simulink model "ch5example2"  (Simulink 5.0)
settings: Solver=ode5  StartTime=0.0  StopTime=0.02  FixedStep=6.23e-8  RelTol=1e-3
values from neighbouring files (symbols this model uses):
  sigma2 = P/SNR_in(k)    [ch5example2prg1.m]
libraries: dsparch4 x6, dspbuff3 x1, dspstat3 x1, dspmathops x1
settings Model: LastModifiedBy=shaoyubin

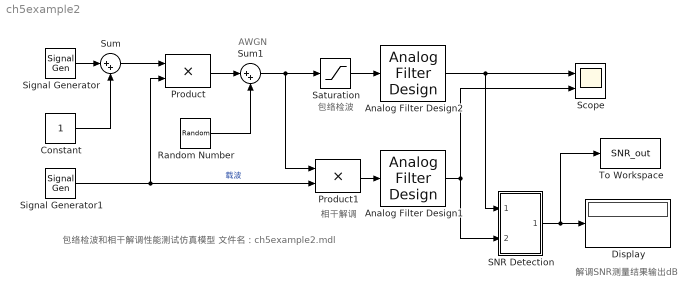
== system ch5example2 ==
  note: 包络检波和相干解调性能测试仿真模型
      | 文件名：ch5example2.mdl
  note: AWGN
  note: 解调SNR测量结果输出dB
  note: 包络检波
  note: 相干解调
  Analog Filter Design1 : dsparch4/Analog Filter Design  method=Butterworth  filttype=Lowpass  N=2  Wlo=2*pi*6e3  Whi=80  Rp=2  Rs=40
  Analog Filter Design2 : dsparch4/Analog Filter Design  method=Butterworth  filttype=Lowpass  N=2  Wlo=2*pi*6e3  Whi=80  Rp=2  Rs=40
  Constant : Constant
  Display : Display
  Product : Product  SaturateOnIntegerOverflow=on
  Product1 : Product  SaturateOnIntegerOverflow=on
  Random Number : RandomNumber  Variance=sigma2  SampleTime=6.23e-8
  SNR Detection : Subsystem
  Saturation : Saturate  UpperLimit=inf  LowerLimit=0
  Scope : Scope  NumInputPorts=2
      settings: TimeRange=0.005  YMin=0~0  YMax=1~1
  Signal Generator : SignalGenerator  Amplitude=0.3*1  Frequency=1000
  Signal Generator1 : SignalGenerator  Frequency=1000e3
  Sum : Sum  Inputs=|++  SaturateOnIntegerOverflow=on
  Sum1 : Sum  Inputs=|++  SaturateOnIntegerOverflow=on
  To Workspace : ToWorkspace  VariableName=SNR_out  SampleTime=-1  SaveFormat=Array
      settings: MaxDataPoints=1
  wires:
  Constant/1 -> Sum/2
  Signal Generator/1 -> Sum/1
  Sum/1 -> Product/1
  Signal Generator1/1 -> Product/2, Product1/2  "载波"
  Product/1 -> Sum1/1
  Random Number/1 -> Sum1/2
  Sum1/1 -> Saturation/1, Product1/1
  Saturation/1 -> Analog Filter Design2/1
  Analog Filter Design2/1 -> SNR Detection/1(In1), Scope/1
  Product1/1 -> Analog Filter Design1/1
  Analog Filter Design1/1 -> SNR Detection/2(In2), Scope/2
  SNR Detection/1(Out1) -> Display/1, To Workspace/1

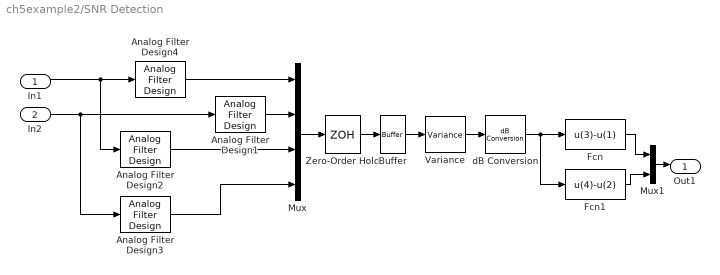
== system ch5example2/SNR Detection ==
  In1 : Inport
  In2 : Inport  Port=2
  Analog Filter Design1 : dsparch4/Analog Filter Design  method=Butterworth  filttype=Bandstop  N=2  Wlo=2*pi*(1e3-100)  Whi=2*pi*(1e3+100)  Rp=2  Rs=40
  Analog Filter Design2 : dsparch4/Analog Filter Design  method=Butterworth  filttype=Bandpass  N=2  Wlo=2*pi*(1e3-100)  Whi=2*pi*(1e3+100)  Rp=2  Rs=40
  Analog Filter Design3 : dsparch4/Analog Filter Design  method=Butterworth  filttype=Bandpass  N=2  Wlo=2*pi*(1e3-100)  Whi=2*pi*(1e3+100)  Rp=2  Rs=40
  Analog Filter Design4 : dsparch4/Analog Filter Design  method=Butterworth  filttype=Bandstop  N=2  Wlo=2*pi*(1e3-100)  Whi=2*pi*(1e3+100)  Rp=2  Rs=40
  Buffer : dspbuff3/Buffer  N=1.6051e+005  V=0  ic=0
  Fcn : Fcn  Expr=u(3)-u(1)
  Fcn1 : Fcn  Expr=u(4)-u(2)
  Mux : Mux
  Mux1 : Mux  Inputs=2
  Variance : dspstat3/Variance  run=off  reset_popup=None
  Zero-Order Hold : ZeroOrderHold  SampleTime=6.23e-8
  dB Conversion : dspmathops/dB Conversion  dBtype=dB  intype=Power  R=1  fuzz=on
  Out1 : Outport
  wires:
  Zero-Order Hold/1 -> Buffer/1
  Variance/1 -> dB Conversion/1
  Mux/1 -> Zero-Order Hold/1
  In1/1 -> Analog Filter Design4/1, Analog Filter Design2/1
  In2/1 -> Analog Filter Design1/1, Analog Filter Design3/1
  Analog Filter Design4/1 -> Mux/1
  Analog Filter Design2/1 -> Mux/3
  Analog Filter Design3/1 -> Mux/4
  Fcn/1 -> Mux1/1
  Buffer/1 -> Variance/1
  dB Conversion/1 -> Fcn/1, Fcn1/1
  Fcn1/1 -> Mux1/2
  Mux1/1 -> Out1/1
  Analog Filter Design1/1 -> Mux/2
